simulink model "lab2_first_part"  (R2022a)
settings: Solver=VariableStepAuto  StartTime=0.0  StopTime=10.0  RelTol=1e-3
settings Model: Creator=Даниил  LastModifiedBy=Даниил

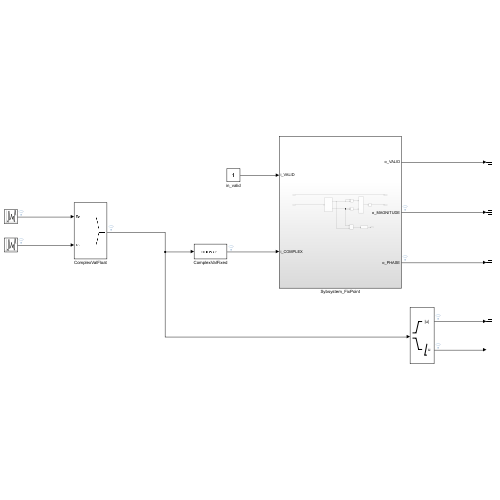
[thumbnail: Simulink's stored preview of the top-level diagram]
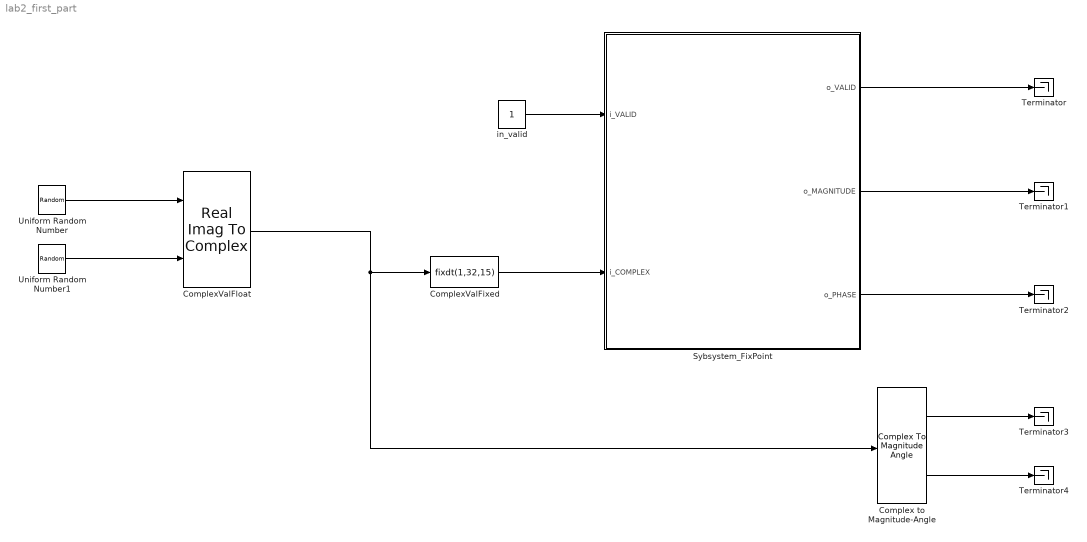
== system lab2_first_part ==
  Complex to Magnitude-Angle : ComplexToMagnitudeAngle
  ComplexValFixed : DataTypeConversion  OutDataTypeStr=fixdt(1,32,15)  RndMeth=Round  SaturateOnIntegerOverflow=off
  ComplexValFloat : RealImagToComplex
  Sybsystem_FixPoint : Subsystem
  Terminator{,1..4} (5 alike) : Terminator
  Uniform Random Number : UniformRandomNumber  Minimum=-2 ^(17 - 1)  Maximum=2 ^(17-1) - 1  Seed=17  SampleTime=1
  Uniform Random Number1 : UniformRandomNumber  Minimum=-2 ^(17 - 1)  Maximum=2 ^(17-1) - 1  Seed=18  SampleTime=1
  in_valid : Constant  OutDataTypeStr=boolean  SampleTime=1
  wires:
  ComplexValFixed/1 -> Sybsystem_FixPoint/2(i_COMPLEX)
  in_valid/1 -> Sybsystem_FixPoint/1(i_VALID)
  ComplexValFloat/1 -> Complex to Magnitude-Angle/1, ComplexValFixed/1
  Complex to Magnitude-Angle/1 -> Terminator3/1
  Complex to Magnitude-Angle/2 -> Terminator4/1
  Sybsystem_FixPoint/3(o_PHASE) -> Terminator2/1
  Sybsystem_FixPoint/2(o_MAGNITUDE) -> Terminator1/1
  Uniform Random Number1/1 -> ComplexValFloat/2
  Uniform Random Number/1 -> ComplexValFloat/1
  Sybsystem_FixPoint/1(o_VALID) -> Terminator/1

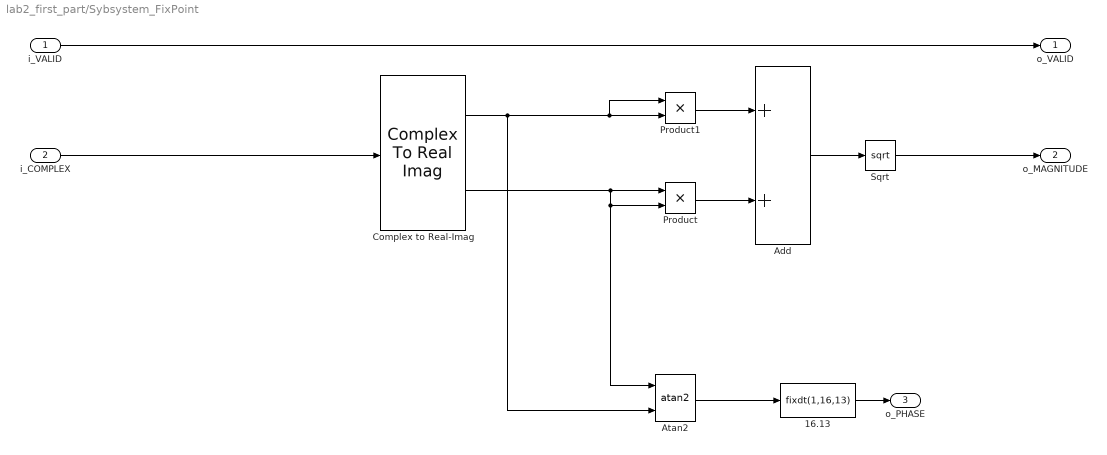
== system lab2_first_part/Sybsystem_FixPoint ==
  i_VALID : Inport  OutDataTypeStr=boolean
  i_COMPLEX : Inport  Port=2
  16.13 : DataTypeConversion  OutDataTypeStr=fixdt(1,16,13)  RndMeth=Round  SaturateOnIntegerOverflow=off
  Add : Sum
  Atan2 : Trigonometry  Operator=atan2  ApproximationMethod=CORDIC
  Complex to Real-Imag : ComplexToRealImag
  Product : Product
  Product1 : Product
  Sqrt : Sqrt  OutDataTypeStr=fixdt(1,33,15)
  o_VALID : Outport
  o_MAGNITUDE : Outport  Port=2
  o_PHASE : Outport  Port=3
  wires:
  Add/1 -> Sqrt/1
  Product1/1 -> Add/1
  Sqrt/1 -> o_MAGNITUDE/1
  Product/1 -> Add/2
  Atan2/1 -> 16.13/1
  i_COMPLEX/1 -> Complex to Real-Imag/1
  i_VALID/1 -> o_VALID/1
  16.13/1 -> o_PHASE/1
  Complex to Real-Imag/2 -> Atan2/1, Product/2, Product/1
  Complex to Real-Imag/1 -> Product1/1, Product1/2, Atan2/2
